simulink model "untitled10"  (R2024a)
settings: Solver=FixedStepAuto  StartTime=0.0  StopTime=10.0  RelTol=1e-3
libraries: androidsensorlib x2, androidaudiovideolib x1, androidcommunicationlib x1
settings Model: Creator=bhand  LastModifiedBy=Prashant Mahawar
settings OptimizationCC: DefaultParameterBehavior=Inlined  EnhancedBackFolding=on  PassReuseOutputArgsAs=Individual arguments  ZeroExternalMemoryAtStartup=off  ZeroInternalMemoryAtStartup=off  MaxStackSize=64  OptimizeBlockOrder=speed  DifferentSizesBufferReuse=on  OptimizationCustomize=off  EfficientTunableParamExpr=on
settings DebuggingCC: ParameterTunabilityLossMsg=error
settings HardwareCC: ProdBitPerLong=64  ProdLargestAtomicInteger=LongLong  ProdLargestAtomicFloat=Double  ProdLongLongMode=on  ProdHWDeviceType=ARM Compatible->ARM Cortex-A (64-bit)  UseEmbeddedCoderFeatures=off  UseSimulinkCoderFeatures=off
settings SFSimCC: MATLABDynamicMemAlloc=off
settings RTWCC: Description=Embedded Coder  SystemTargetFile=ert.tlc  HardwareBoard=Android Device (64bit)  TLCOptions="-aInlineSetEventsForThisBaseRateFcn=TLC_FALSE -aSuppressMultiTaskScheduler=TLC_FALSE  -aRateBasedStepFcn=0"  TemplateMakefile=ert_default_tmf  RTWVerbose=off  Toolchain=Android SDK/NDK Tools
settings CodeAppCC: ForceParamTrailComments=on  IgnoreCustomStorageClasses=off  OperatorAnnotations=on  SimulinkDataObjDesc=on  SFDataObjDesc=on  InsertBlockDesc=on
settings ERTTargetCC: SupportNonInlinedSFcns=on  InlinedParameterPlacement=NonHierarchical

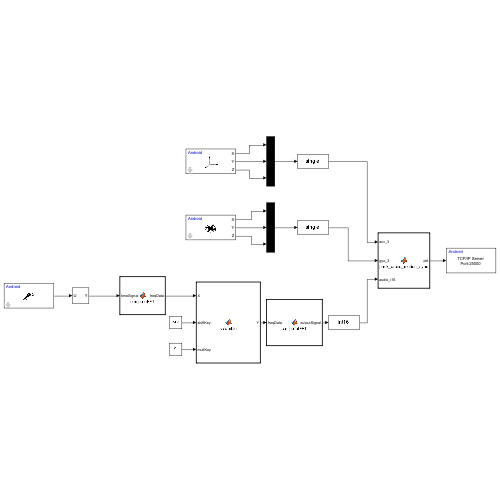
[thumbnail: Simulink's stored preview of the top-level diagram]
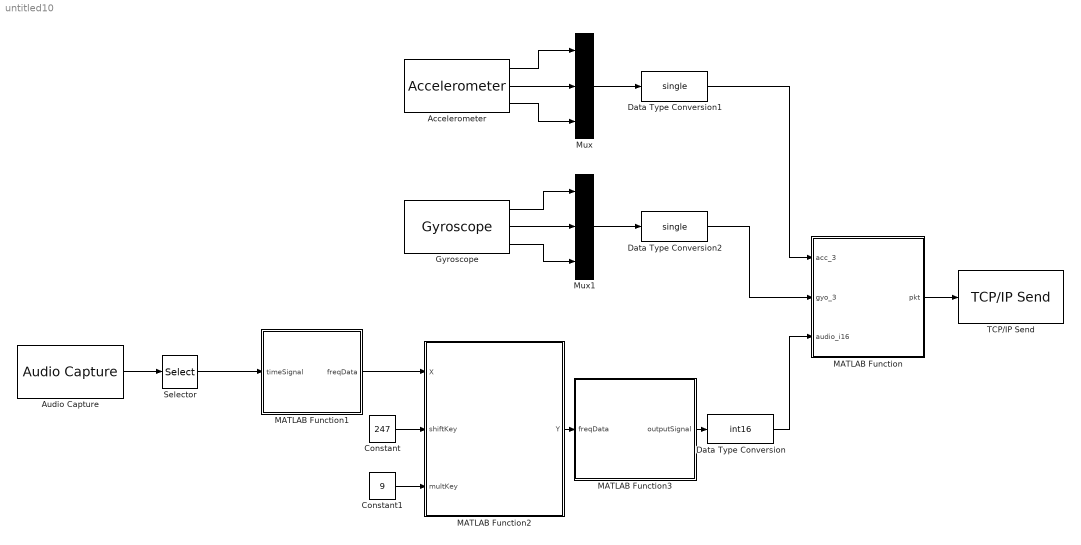
== system untitled10 ==
  Accelerometer : androidsensorlib/Accelerometer  OutputVector=off  SampleTime=0.1  BlockPlatform=Android
  Audio Capture : androidaudiovideolib/Audio Capture  SampleFreq=44100  FrameSize=4410  SampleTime=0.1  SimulateUsing=Code generation  DeviceStr=0  QueueDuration=0  BlockPlatform=Android  AudioSamplingFreq=44100
  Constant : Constant  Value=247
  Constant1 : Constant  Value=9
  Data Type Conversion : DataTypeConversion  OutDataTypeStr=int16  SaturateOnIntegerOverflow=off  RndMeth=Floor
  Data Type Conversion1 : DataTypeConversion  OutDataTypeStr=single  SaturateOnIntegerOverflow=off  RndMeth=Floor
  Data Type Conversion2 : DataTypeConversion  OutDataTypeStr=single  SaturateOnIntegerOverflow=off  RndMeth=Floor
  Gyroscope : androidsensorlib/Gyroscope  OutputVector=off  SampleTime=0.1  BlockPlatform=Android
  MATLAB Function : MATLAB Function  TreatAsAtomicUnit=on
  MATLAB Function1 : MATLAB Function  TreatAsAtomicUnit=on
  MATLAB Function2 : MATLAB Function  TreatAsAtomicUnit=on
  MATLAB Function3 : MATLAB Function  TreatAsAtomicUnit=on
  Mux : Mux  Inputs=3
  Mux1 : Mux  Inputs=3
  Selector : Selector  NumberOfDimensions=2  InputPortWidth=3  IndexOptions=Select all,Index vector (dialog)  Indices=[1 3],1  OutputSizes=1,1
  TCP/IP Send : androidcommunicationlib/TCP//IP Send  TCPSendId=untitled10/TCP//IP_Send  Mode_=Server  LocalServerPort_=25000  RemoteAddr_=127.0.0.1  RemoteServerPort_=25000  ClientPortBindingSelection_=off  ClientPortToBind_=35000  BlockingMode_=off  BlockTimeout_=0.1
  wires:
  Constant/1 -> MATLAB Function2/2(shiftKey)
  MATLAB Function1/1(freqData) -> MATLAB Function2/1(X)
  Audio Capture/1 -> Selector/1
  MATLAB Function2/1(Y) -> MATLAB Function3/1(freqData)
  Accelerometer/1 -> Mux/1
  Gyroscope/2 -> Mux1/2
  Gyroscope/3 -> Mux1/3
  Accelerometer/2 -> Mux/2
  Mux/1 -> Data Type Conversion1/1
  Gyroscope/1 -> Mux1/1
  Accelerometer/3 -> Mux/3
  MATLAB Function/1(pkt) -> TCP/IP Send/1
  Data Type Conversion1/1 -> MATLAB Function/1(acc_3)
  Data Type Conversion/1 -> MATLAB Function/3(audio_i16)
  Selector/1 -> MATLAB Function1/1(timeSignal)
  MATLAB Function3/1(outputSignal) -> Data Type Conversion/1
  Mux1/1 -> Data Type Conversion2/1
  Constant1/1 -> MATLAB Function2/3(multKey)
  Data Type Conversion2/1 -> MATLAB Function/2(gyo_3)

== matlab function untitled10/MATLAB Function1 ==
  data: timeSignal input; freqData output
function freqData = computeFFT(timeSignal)
% Verify input is a vector
assert(isvector(timeSignal), 'computeFFT: timeSignal must be a vector.');

% Track input orientation (row or column)
inputWasRow = isrow(timeSignal);

% Convert input to single precision column vector
timeSignal = single(timeSignal(:));
numSamples = length(timeSignal);

% Perform FFT and normalize to prevent amplitude scaling
freqData = fft(timeSignal) / single(numSamples);

% Preserve the input shape
if inputWasRow
    freqData = freqData.';
end
end

== matlab function untitled10/MATLAB Function3 ==
  data: freqData input; outputSignal output
function outputSignal = computeIFFT(freqData)

% Ensure input is a vector
assert(isvector(freqData), 'computeIFFT: freqData must be a vector.');

% Check orientation (row or column)
inputWasRow = isrow(freqData);

% Convert input to a complex single-precision column vector
freqData = complex(single(freqData(:)));
numPts = length(freqData);

% Perform IFFT (multiply by N to undo FFT normalization)
tempResult = ifft(freqData * single(numPts));

% Extract the real part of the signal
outputSignal = real(tempResult);

% Preserve original shape
if inputWasRow
    outputSignal = outputSignal.';
end
end

== matlab function untitled10/MATLAB Function2 ==
  data: X input; Y output; shiftKey input; multKey input
function Y = scramble(X, shiftKey, multKey)
%#codegen
% scramble - Shifts frequency bins and scales magnitude.
%
% Inputs:
%   X         : Frequency domain input (vector)
%   shiftKey  : Number of bins to right-shift
%   multKey   : Scalar multiplier for magnitude
%
% Output:
%   Y         : Scrambled output after shift and magnitude scaling

% Ensure input is a vector
assert(isvector(X), 'Input must be a vector.');

% Make sure keys are numeric
shiftKey = double(shiftKey);
multKey  = double(multKey);

% Step 1: Circularly shift the frequency bins
Y = circshift(X, shiftKey);

% Step 2: Multiply the magnitude of the frequency bins
Y = abs(Y) * multKey .* exp(1j * angle(Y));

end

== matlab function untitled10/MATLAB Function ==
  data: acc_3 input size=6; gyo_3 input; pkt output size=8848; audio_i16 input size=4410
function pkt = pack_audio_motion_sync(acc_3, gyo_3, audio_i16)
%#codegen
persistent t;
if isempty(t)
    t = uint32(0);
end
t = t + uint32(1);
%Each time the value of t increases by 1 which can be considered to be 0.1s 

% Converting to bytes and ensuring column orientation
time_bytes   = reshape(typecast(t,        'uint8'), [], 1); % 4×1
acc_bytes = reshape(typecast(acc_3,  'uint8'), [], 1); % 12×1
gyo_bytes = reshape(typecast(gyo_3,  'uint8'), [], 1); % 12×1
audio_bytes  = reshape(typecast(audio_i16,'uint8'), [], 1); % 8820×1

% Concatenating: total 8848×1 length
pkt = [time_bytes; acc_bytes; gyo_bytes; audio_bytes];
end
